simulink model "q1"  (Simulink 6.6)
settings: Solver=ode45  StartTime=0.0  StopTime=10.0  RelTol=1e-3
InitFcn:
  | R1 = 40000;
  | R2 = 60000;
  | 
  | K = 0.5;
  | 
  | C1= 0.000000250;
  | C2= C1;
libraries: simulink_extras x1
settings Model: Creator=Johnny  LastModifiedBy=Johnny

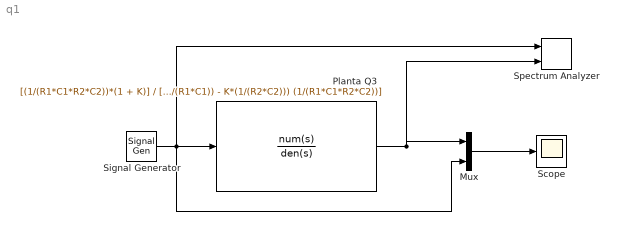
== system q1 ==
  Mux : Mux  Inputs=2
  Planta Q3 : TransferFcn  Numerator=[(1/(R1*C1*R2*C2))*(1 + K)]  Denominator=[1 ((1/(R2*C1)) + (1/(R1*C1)) - K*(1/(R2*C2))) (1/(R1*C1*R2*C2))]
  Scope : Scope
  Signal Generator : SignalGenerator  WaveForm=square  Frequency=2  Units=rad/sec
  Spectrum Analyzer : simulink_extras/Additional Sinks/Spectrum Analyzer  SystemSampleTime=-1  npts=256  fftpts=256  HowOften=64  sampleT=0.1
  wires:
  Signal Generator/1 -> Planta Q3/1, Spectrum Analyzer/1, Mux/2
  Planta Q3/1 -> Spectrum Analyzer/2, Mux/1
  Mux/1 -> Scope/1
